simulink model "prove_import"  (R2018b)
settings: Solver=VariableStepAuto  StartTime=0.0  StopTime=10.0  RelTol=1e-3
settings Model: Creator=Utente  LastModifiedBy=Utente

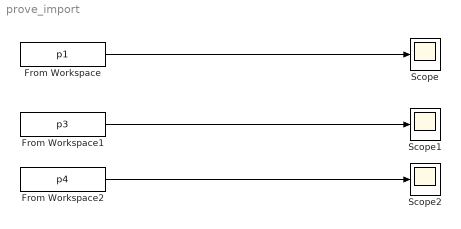
== system prove_import ==
  From Workspace : FromWorkspace  VariableName=p1  SampleTime=0
  From Workspace1 : FromWorkspace  VariableName=p3  SampleTime=0
  From Workspace2 : FromWorkspace  VariableName=p4  SampleTime=0
  Scope : Scope
  Scope1 : Scope
  Scope2 : Scope
  wires:
  From Workspace/1 -> Scope/1
  From Workspace1/1 -> Scope1/1
  From Workspace2/1 -> Scope2/1
